simulink model "Factorial"  (R2021a)
settings: Solver=VariableStepAuto  StartTime=0.0  StopTime=1  RelTol=1e-3  EnableMultiTasking=on
settings Model: Creator=pc  LastModifiedBy=pc
settings SolverCC: AlgebraicLoopSolver=TrustRegion
settings DataIOCC: ReturnWorkspaceOutputs=off
settings OptimizationCC: LifeSpan=inf
settings DebuggingCC: SFUnexpectedBacktrackingDiag=warning  SFNoUnconditionalDefaultTransitionDiag=warning  SFMachineParentedDataDiag=warning  ArithmeticOperatorsInVariantConditions=warning
settings SFSimCC: SimUseLocalCustomCode=off  CustomCodeUndefinedFunction=UseInterfaceOnly
settings RTWCC: RTWUseLocalCustomCode=off
settings CodeAppCC: StateflowObjectComments=on
settings GRTTargetCC: TargetLangStandard=C89/C90 (ANSI)
settings ConfigComp: CovMetricSettings=dw  CovSaveCumulativeToWorkspaceVar=on  CovSaveSingleToWorkspaceVar=on  CovExternalEMLEnable=off
settings SimscapeCC: SimscapeNormalizeSystem=off

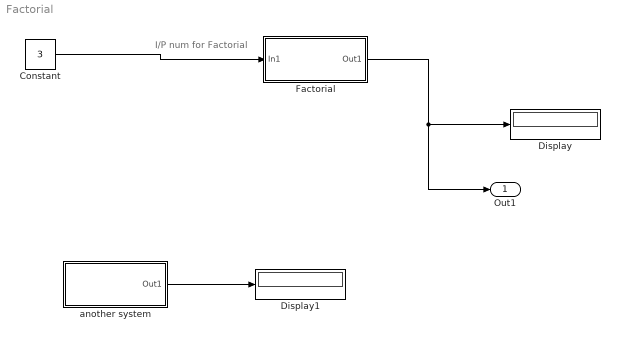
== system Factorial ==
  note: I/P num for Factorial
  Constant : Constant  Value=3  OutDataTypeStr=int32  SampleTime=-1
  Display : Display
  Display1 : Display
  Factorial : Subsystem  TreatAsAtomicUnit=on
  another system : Subsystem  TreatAsAtomicUnit=on
  Out1 : Outport  OutDataTypeStr=int32
  wires:
  Factorial/1(Out1) -> Display/1, Out1/1
  Constant/1 -> Factorial/1(In1)
  another system/1(Out1) -> Display1/1

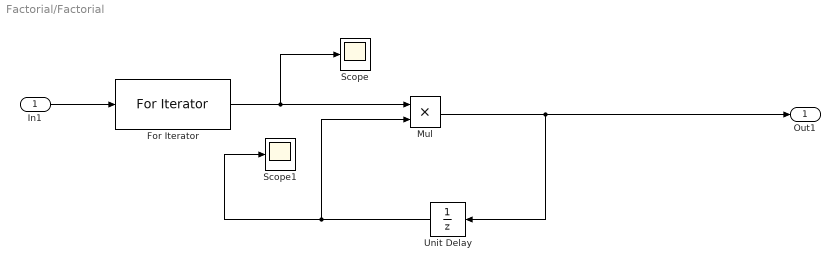
== system Factorial/Factorial ==
  In1 : Inport  OutDataTypeStr=int32
  For Iterator : ForIterator  ResetStates=reset  IterationSource=external
  Mul : Product  OutDataTypeStr=Inherit: Same as first input
  Scope : Scope
  Scope1 : Scope
  Unit Delay : UnitDelay  InitialCondition=1  SampleTime=-1  HasFrameUpgradeWarning=on
  Out1 : Outport  OutDataTypeStr=int32
  wires:
  In1/1 -> For Iterator/1
  For Iterator/1 -> Scope/1, Mul/1
  Mul/1 -> Unit Delay/1, Out1/1
  Unit Delay/1 -> Scope1/1, Mul/2

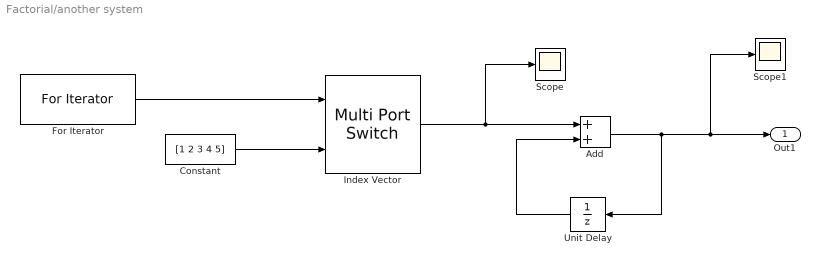
== system Factorial/another system ==
  Add : Sum
  Constant : Constant  Value=[1 2 3 4 5]
  For Iterator : ForIterator  ResetStates=reset  IndexMode=Zero-based
  Index Vector : MultiPortSwitch  DataPortOrder=Zero-based contiguous  Inputs=1  zeroidx=on
  Scope : Scope
  Scope1 : Scope
  Unit Delay : UnitDelay  SampleTime=-1  HasFrameUpgradeWarning=on
  Out1 : Outport
  wires:
  For Iterator/1 -> Index Vector/1
  Constant/1 -> Index Vector/2
  Index Vector/1 -> Scope/1, Add/1
  Unit Delay/1 -> Add/2
  Add/1 -> Unit Delay/1, Scope1/1, Out1/1
